simulink model "Fig233"  (R2014a)
settings: Solver=ode3  StartTime=0.0  StopTime=.005  FixedStep=2e-5  RelTol=1e-3
libraries: commfilt2 x1
settings Model: Creator=Dennis Silage  LastModifiedBy=Silage
settings DataIOCC: SignalLoggingSaveFormat=ModelDataLogs
settings OptimizationCC: ExpressionDepthLimit=2147483647  InitFltsAndDblsToZero=on
settings DebuggingCC: UnderspecifiedInitializationDetection=Classic  FcnCallInpInsideContextMsg=UseLocalSettings  StateNameClashWarn=warning  StrictBusMsg=Warning
settings GRTTargetCC: CombineOutputUpdateFcns=off  GRTInterface=on

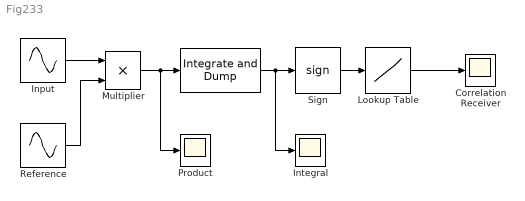
== system Fig233 ==
  " " : commfilt2/Integrate and Dump  obssamples=50  offsetsamples=0  nodump=off  roundingMode=Floor  overflowMode=off
  Correlation Receiver : Scope
      settings: YMin=0  YMax=30
  Input : Sin  Frequency=3141.59  SampleTime=20e-6  VectorParams1D=off
  Integral : Scope
      settings: YMin=0  YMax=1.5  SaveName=ScopeData2
  Lookup Table : Lookup  InputValues=[-1,0,1]  Table=[-1,-1,1]
  Multiplier : Product  RndMeth=Zero
  Product : Scope
      settings: YMin=0  YMax=1.5
  Reference : Sin  Frequency=3141.5926  SampleTime=20e-6
  Sign : Signum
  wires:
  Multiplier/1 -> " "/1, Product/1
  Input/1 -> Multiplier/1
  Reference/1 -> Multiplier/2
  Sign/1 -> Lookup Table/1
  " "/1 -> Sign/1, Integral/1
  Lookup Table/1 -> Correlation Receiver/1
